simulink model "R3_double"  (R2014b)
settings: Solver=ode3  SolverMode=SingleTasking  StartTime=0.0  StopTime=Tsim  FixedStep=Ts  RelTol=1e-3
InitFcn:
  | configDoubleIntegrator
libraries: simulink x1
settings Model: CovMetricSettings=dwe  CovHtmlReporting=off  covSaveCumulativeToWorkspaceVar=off  CovSaveSingleToWorkspaceVar=off  CovExternalEMLEnable=on  CovSFcnEnable=on  Creator=mnade  LastModifiedBy=nina
settings DataIOCC: LimitDataPoints=off  SaveFormat=StructureWithTime
settings DebuggingCC: SolverPrmCheckMsg=none  FrameProcessingCompatibilityMsg=error  SFUnexpectedBacktrackingDiag=error  SFNoUnconditionalDefaultTransitionDiag=error
settings HardwareCC: ProdBitPerPointer=64  ProdLargestAtomicFloat=Float  ProdIntDivRoundTo=Zero  ProdEndianess=LittleEndian  ProdHWDeviceType=Specified
settings ModelReferenceCC: PropagateSignalLabelsOutOfModel=on
settings GRTTargetCC: TargetLangStandard=C99 (ISO)  GeneratePreprocessorConditionals=Use local settings

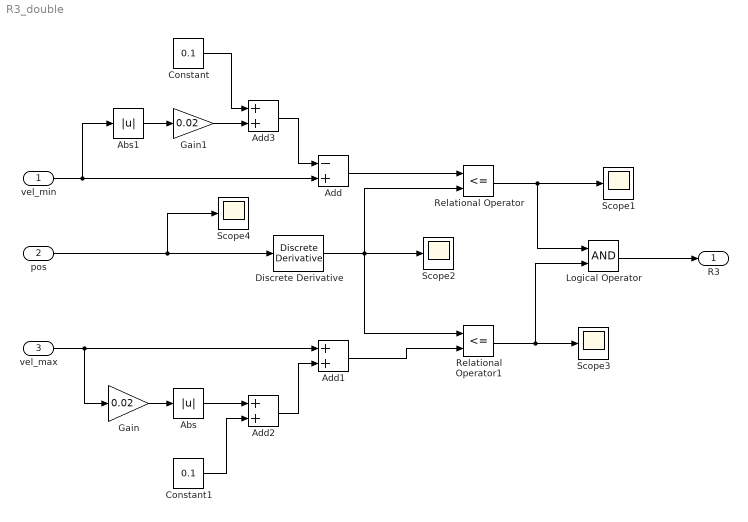
== system R3_double ==
  vel_min : Inport
  pos : Inport  Port=2
  vel_max : Inport  Port=3
  Abs : Abs
  Abs1 : Abs
  Add : Sum  Inputs=-+
  Add1 : Sum
  Add2 : Sum
  Add3 : Sum
  Constant : Constant  Value=0.1
  Constant1 : Constant  Value=0.1
  Discrete Derivative : simulink/Discrete/Discrete Derivative  gainval=1.0  ICPrevScaledInput=0.0  InputProcessing=Inherited  OutMin=[]  OutMax=[]  OutDataType=fixdt(1, 16)  OutScaling=2^-10  DoSatur=off
  Gain : Gain  Gain=0.02
  Gain1 : Gain  Gain=0.02
  Logical Operator : Logic  AllPortsSameDT=off  OutDataTypeStr=boolean
  Relational Operator : RelationalOperator  Operator=<=  OutDataTypeStr=boolean
  Relational Operator1 : RelationalOperator  Operator=<=  OutDataTypeStr=boolean
  Scope{1..4} (4 alike) : Scope
      Scope3 settings: SaveName=ScopeData3
      Scope4 settings: SaveName=ScopeData2
  R3 : Outport
  wires:
  pos/1 -> Discrete Derivative/1, Scope4/1
  Discrete Derivative/1 -> Scope2/1, Relational Operator1/1, Relational Operator/2
  Relational Operator/1 -> Scope1/1, Logical Operator/1
  Logical Operator/1 -> R3/1
  vel_min/1 -> Abs1/1, Add/2
  vel_max/1 -> Gain/1, Add1/1
  Relational Operator1/1 -> Scope3/1, Logical Operator/2
  Gain/1 -> Abs/1
  Gain1/1 -> Add3/2
  Add/1 -> Relational Operator/1
  Add1/1 -> Relational Operator1/2
  Abs/1 -> Add2/1
  Abs1/1 -> Gain1/1
  Add2/1 -> Add1/2
  Add3/1 -> Add/1
  Constant/1 -> Add3/1
  Constant1/1 -> Add2/2
